simulink model "Deadlockv2"  (R2025a)
settings: Solver=FixedStepDiscrete  StartTime=0.0  StopTime=60  FixedStep=.1  RelTol=1e-3
undefined symbols (not defined in the file or in its folder): DiscIntNeverNeededParam
libraries: simulink x2
settings Model: Creator=nirmay  LastModifiedBy=nirmay

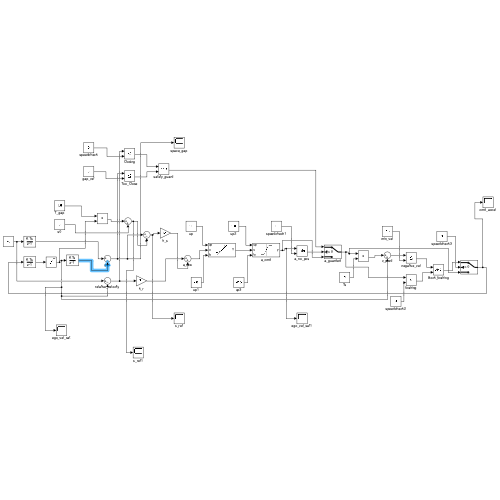
[thumbnail: Simulink's stored preview of the top-level diagram]
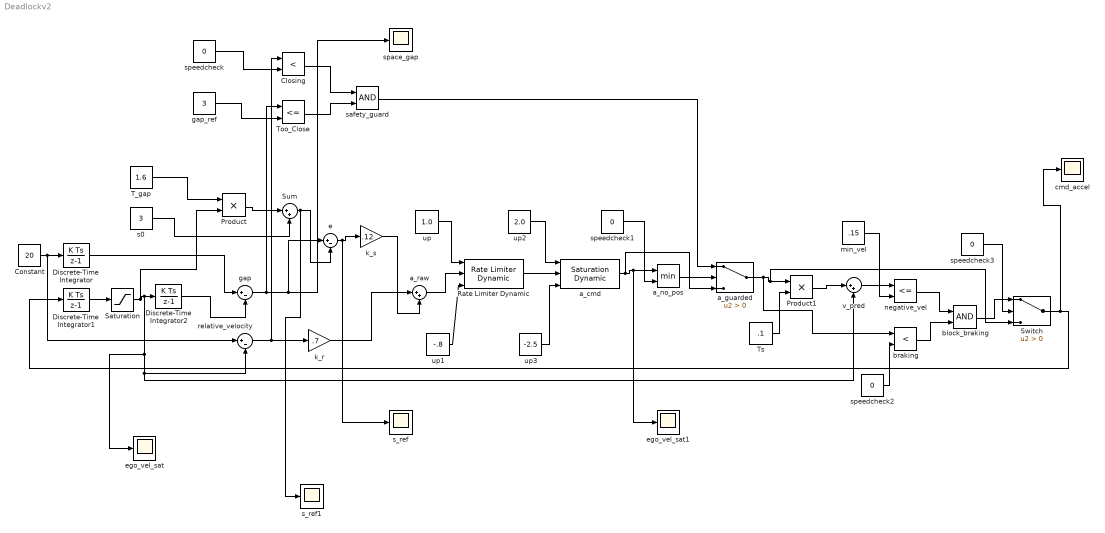
== system Deadlockv2 ==
  Closing : RelationalOperator  Operator=<  OutDataTypeStr=boolean  RndMeth=Simplest  InputSameDT=off
  Constant : Constant  Value=20  SampleTime=.1
  Discrete-Time Integrator : DiscreteIntegrator  InitialCondition=40  SampleTime=-1  ICPrevOutput=DiscIntNeverNeededParam  ICPrevScaledInput=DiscIntNeverNeededParam
  Discrete-Time Integrator1 : DiscreteIntegrator  SampleTime=-1  ICPrevOutput=DiscIntNeverNeededParam  ICPrevScaledInput=DiscIntNeverNeededParam
  Discrete-Time Integrator2 : DiscreteIntegrator  SampleTime=-1  ICPrevOutput=DiscIntNeverNeededParam  ICPrevScaledInput=DiscIntNeverNeededParam
  Product : Product
  Product1 : Product
  Rate Limiter Dynamic : simulink/Discontinuities/Rate Limiter Dynamic
  Saturation : Saturate  UpperLimit=inf  LowerLimit=0
  Sum : Sum  Inputs=|++
  Switch : Switch  Criteria=u2 > Threshold  SaturateOnIntegerOverflow=off  InputSameDT=off
  T_gap : Constant  Value=1.6  SampleTime=.1
  Too_Close : RelationalOperator  Operator=<=  OutDataTypeStr=boolean  RndMeth=Simplest  InputSameDT=off
  Ts : Constant  Value=.1  SampleTime=.1
  a_cmd : simulink/Discontinuities/Saturation Dynamic  OutMin=[]  OutMax=[]  OutDataTypeStr=Inherit: Same as second input  OutDataType=fixdt(1, 16)  OutScaling=2^-10  DoSatur=off
  a_guarded : Switch  Criteria=u2 > Threshold  SaturateOnIntegerOverflow=off  InputSameDT=off
  a_no_pos : MinMax  Inputs=2
  a_raw : Sum  Inputs=|++
  block_braking : Logic  AllPortsSameDT=off  OutDataTypeStr=boolean
  braking : RelationalOperator  Operator=<  OutDataTypeStr=boolean  RndMeth=Simplest  InputSameDT=off
  cmd_accel : Scope
      settings: ActiveDisplayYMinimum=-3.0625  ActiveDisplayYMaximum=2.5625
  e : Sum  Inputs=|+-
  ego_vel_sat : Scope
      settings: ActiveDisplayYMinimum=-1  ActiveDisplayYMaximum=1  DataLoggingVariableName=ScopeData2
  ego_vel_sat1 : Scope
      settings: ActiveDisplayYMinimum=-1  ActiveDisplayYMaximum=1  DataLoggingVariableName=ScopeData4
  gap : Sum  Inputs=|+-
  gap_ref : Constant  Value=3  SampleTime=.1
  k_r : Gain  Gain=.7
  k_s : Gain  Gain=.12
  min_vel : Constant  Value=.15  SampleTime=.1
  negative_vel : RelationalOperator  Operator=<=  OutDataTypeStr=boolean  RndMeth=Simplest  InputSameDT=off
  relative_velocity : Sum  Inputs=|+-
  s0 : Constant  Value=3  SampleTime=.1
  s_ref : Scope
      settings: ActiveDisplayYMinimum=-600.81804500000612  ActiveDisplayYMaximum=187.20200500000078  DataLoggingVariableName=ScopeData3
  s_ref1 : Scope
      settings: ActiveDisplayYMinimum=-10.864000000000056  ActiveDisplayYMaximum=97.776000000000522  DataLoggingVariableName=ScopeData5
  safety_guard : Logic  AllPortsSameDT=off  OutDataTypeStr=boolean
  space_gap : Scope
      settings: ActiveDisplayYMinimum=-1  ActiveDisplayYMaximum=1
  speedcheck{,1..3} (4 alike) : Constant  Value=0  SampleTime=.1
  up : Constant  Value=1.0  SampleTime=.1
  up1 : Constant  Value=-.8  SampleTime=.1
  up2 : Constant  Value=2.0  SampleTime=.1
  up3 : Constant  Value=-2.5  SampleTime=.1
  v_pred : Sum  Inputs=|++
  wires:
  Constant/1 -> relative_velocity/1, Discrete-Time Integrator/1
  Discrete-Time Integrator2/1 -> gap/2
  Discrete-Time Integrator1/1 -> Saturation/1
  Saturation/1 -> Product/2, ego_vel_sat/1, v_pred/2, relative_velocity/2, Discrete-Time Integrator2/1
  Discrete-Time Integrator/1 -> gap/1
  T_gap/1 -> Product/1
  s0/1 -> Sum/2
  Product/1 -> Sum/1
  gap/1 -> Too_Close/1, space_gap/1, e/1
  Sum/1 -> s_ref1/1, e/2
  e/1 -> s_ref/1, k_s/1
  relative_velocity/1 -> Closing/1, k_r/1
  k_r/1 -> a_raw/1
  k_s/1 -> a_raw/2
  a_raw/1 -> Rate Limiter Dynamic/2
  up/1 -> Rate Limiter Dynamic/1
  up1/1 -> Rate Limiter Dynamic/3
  Rate Limiter Dynamic/1 -> a_cmd/2
  up3/1 -> a_cmd/3
  up2/1 -> a_cmd/1
  gap_ref/1 -> Too_Close/2
  speedcheck/1 -> Closing/2
  Closing/1 -> safety_guard/1
  Too_Close/1 -> safety_guard/2
  a_cmd/1 -> a_guarded/3, ego_vel_sat1/1, a_no_pos/1
  speedcheck1/1 -> a_no_pos/2
  safety_guard/1 -> a_guarded/1
  a_no_pos/1 -> a_guarded/2
  a_guarded/1 -> braking/1, Switch/3, Product1/1
  Ts/1 -> Product1/2
  Product1/1 -> v_pred/1
  v_pred/1 -> negative_vel/1
  min_vel/1 -> negative_vel/2
  speedcheck2/1 -> braking/2
  negative_vel/1 -> block_braking/1
  braking/1 -> block_braking/2
  block_braking/1 -> Switch/1
  speedcheck3/1 -> Switch/2
  Switch/1 -> cmd_accel/1, Discrete-Time Integrator1/1
